simulink model "zadanie2"  (R2020a)
settings: Solver=FixedStepAuto  StartTime=0.0  StopTime=10  FixedStep=0.005  RelTol=1e-3
values from neighbouring files (symbols this model uses):
  A = 2    [zadanie2_skrypt.m]
  w = [1,pi/2,2,pi,5,2*pi,10,20,25,30]    [zadanie2_skrypt.m]
settings Model: Creator=admin  LastModifiedBy=admin

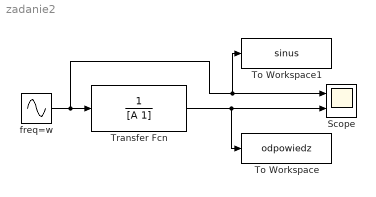
== system zadanie2 ==
  Scope : Scope  NumInputPorts=2
  To Workspace : ToWorkspace  VariableName=odpowiedz  SaveFormat=Timeseries  SampleTime=-1
  To Workspace1 : ToWorkspace  VariableName=sinus  SaveFormat=Timeseries  SampleTime=-1
  Transfer Fcn : TransferFcn  Denominator=[A 1]
  freq=w : Sin  Frequency=w  SampleTime=0
  wires:
  Transfer Fcn/1 -> Scope/2, To Workspace/1
  freq=w/1 -> To Workspace1/1, Scope/1, Transfer Fcn/1
